simulink model "mrac_sim"  (R2023b)
settings: Solver=FixedStepDiscrete  StartTime=0.0  StopTime=6*60  FixedStep=0.1  RelTol=1e-3  EnableMultiTasking=on
undefined symbols (not defined in the file): Advantech, PCI
libraries: sldrtlib x4
settings Model: Creator=Admin  LastModifiedBy=andre
settings SolverCC: AlgebraicLoopSolver=TrustRegion
settings DataIOCC: LimitDataPoints=on  SaveFormat=Array  ReturnWorkspaceOutputs=off
settings OptimizationCC: ReuseModelBlockBuffer=off  LifeSpan=inf
settings DebuggingCC: UnconnectedInputMsg=warning  UnconnectedOutputMsg=warning  UnconnectedLineMsg=warning  SFUnexpectedBacktrackingDiag=warning  SFNoUnconditionalDefaultTransitionDiag=warning  SFExecutionAtInitializationDiag=none  ArithmeticOperatorsInVariantConditions=warning
settings HardwareCC: ProdBitPerPointer=32  ProdBitPerSizeT=32  ProdBitPerPtrDiffT=32  ProdLargestAtomicFloat=None  ProdIntDivRoundTo=Undefined  ProdEndianess=Unspecified  ProdWordSize=32  ProdHWDeviceType=32-bit Generic
settings ModelReferenceCC: PropagateSignalLabelsOutOfModel=off
settings SFSimCC: SimUseLocalCustomCode=off  CustomCodeUndefinedFunction=UseInterfaceOnly
settings RTWCC: RTWUseLocalCustomCode=off
settings CodeAppCC: StateflowObjectComments=on
settings GRTTargetCC: TargetLangStandard=C89/C90 (ANSI)
settings ConfigComp: CovMetricSettings=dw  CovSaveCumulativeToWorkspaceVar=on  CovSaveSingleToWorkspaceVar=on  CovExternalEMLEnable=off

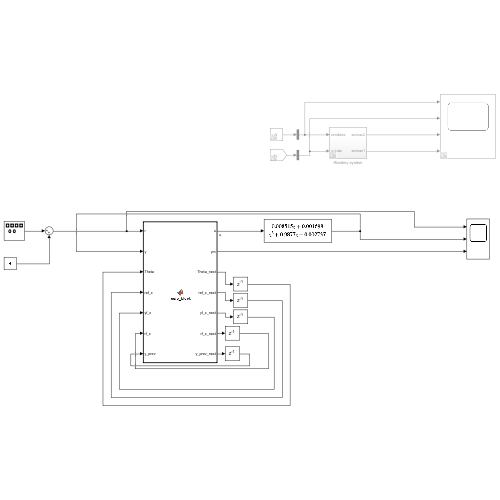
[thumbnail: Simulink's stored preview of the top-level diagram]
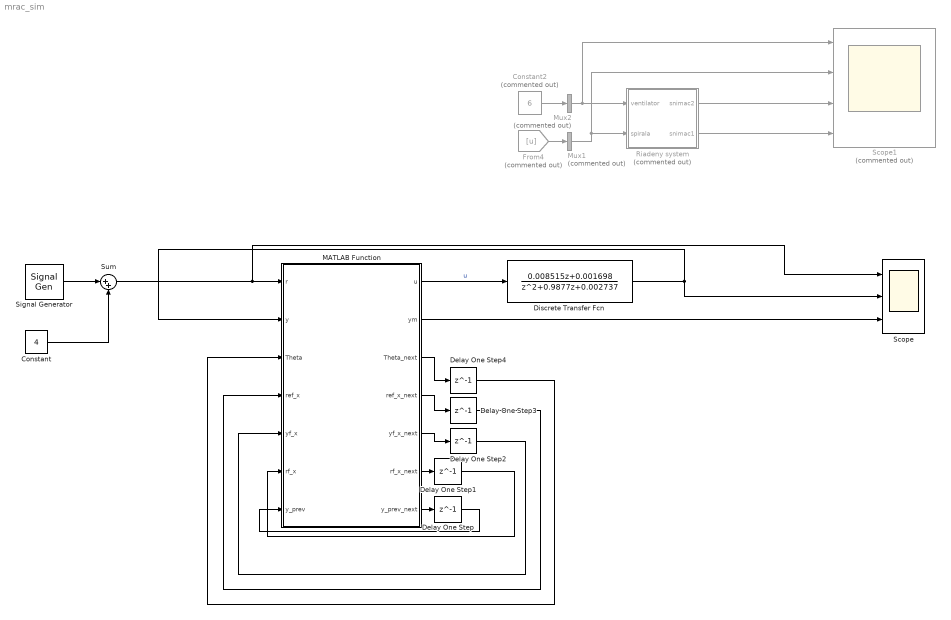
== system mrac_sim ==
  Constant : Constant  Value=4
  Constant2 : Constant  Commented=on  Value=6
  Delay One Step{,1..4} (5 alike) : Delay  DelayLength=1
  Discrete Transfer Fcn : DiscreteTransferFcn  Numerator=[0.008515 0.001698]  Denominator=[1 0.9877 0.002737]
  From4 : From  Commented=on  GotoTag=u
  MATLAB Function : MATLAB Function  TreatAsAtomicUnit=on
  Mux1 : Mux  Commented=on  Inputs=1
  Mux2 : Mux  Commented=on  Inputs=1
  Riadeny system : Subsystem  Commented=on
  Scope : Scope  NumInputPorts=3
  Scope1 : Scope  Commented=on  NumInputPorts=4
  Signal Generator : SignalGenerator  WaveForm=square  Amplitude=2  Frequency=1/50
  Sum : Sum  Inputs=|++
  wires:
  From4/1 -> Mux1/1
  Mux1/1 -> Riadeny system/2(spirala), Scope1/2
  Riadeny system/2(snimac1) -> Scope1/4
  Mux2/1 -> Riadeny system/1(ventilator), Scope1/1
  Riadeny system/1(snimac2) -> Scope1/3
  Constant2/1 -> Mux2/1
  MATLAB Function/7(y_prev_next) -> Delay One Step/1
  MATLAB Function/6(rf_x_next) -> Delay One Step1/1
  MATLAB Function/5(yf_x_next) -> Delay One Step2/1
  MATLAB Function/4(ref_x_next) -> Delay One Step3/1
  MATLAB Function/3(Theta_next) -> Delay One Step4/1
  Sum/1 -> Scope/1, MATLAB Function/1(r)
  Discrete Transfer Fcn/1 -> MATLAB Function/2(y), Scope/2
  MATLAB Function/1(u) -> Discrete Transfer Fcn/1  "u"
  Delay One Step4/1 -> MATLAB Function/3(Theta)
  Delay One Step3/1 -> MATLAB Function/4(ref_x)
  Delay One Step2/1 -> MATLAB Function/5(yf_x)
  Delay One Step1/1 -> MATLAB Function/6(rf_x)
  Delay One Step/1 -> MATLAB Function/7(y_prev)
  Signal Generator/1 -> Sum/1
  Constant/1 -> Sum/2
  MATLAB Function/2(ym) -> Scope/3

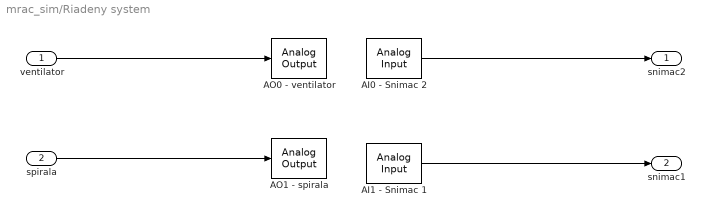
== system mrac_sim/Riadeny system ==
  ventilator : Inport
  spirala : Inport  Port=2
  AI0 - Snimac 2 : sldrtlib/Analog Input  SampleTime=0.1  MaxMissedTicks=10  ShowMissedTicks=off  YieldWhenWaiting=off  DrvName=Advantech/PCI-1711  DrvAddress=4294967295  DrvOptions=zeros(1,0)  Channels=1  RangeMode=1  VoltRange=1  DataType=1
      settings: AttributesFormatString=Advantech\nPCI-1711 [auto]
  AI1 - Snimac 1 : sldrtlib/Analog Input  SampleTime=0.1  MaxMissedTicks=10  ShowMissedTicks=off  YieldWhenWaiting=off  DrvName=Advantech/PCI-1711  DrvAddress=4294967295  DrvOptions=zeros(1,0)  Channels=2  RangeMode=1  VoltRange=1  DataType=1
      settings: AttributesFormatString=Advantech\nPCI-1711 [auto]
  AO0 - ventilator : sldrtlib/Analog Output  SampleTime=0.1  MaxMissedTicks=10  ShowMissedTicks=off  YieldWhenWaiting=off  DrvName=Advantech/PCI-1711  DrvAddress=4294967295  DrvOptions=zeros(1,0)  Channels=1  RangeMode=1  VoltRange=2  InitialValue=[]  FinalValue=[]
      settings: AttributesFormatString=Advantech\nPCI-1711 [auto]
  AO1 - spirala : sldrtlib/Analog Output  SampleTime=0.1  MaxMissedTicks=10  ShowMissedTicks=off  YieldWhenWaiting=off  DrvName=Advantech/PCI-1711  DrvAddress=4294967295  DrvOptions=zeros(1,0)  Channels=2  RangeMode=1  VoltRange=2  InitialValue=[]  FinalValue=[]
      settings: AttributesFormatString=Advantech\nPCI-1711 [auto]
  snimac2 : Outport
  snimac1 : Outport  Port=2
  wires:
  ventilator/1 -> AO0 - ventilator/1
  spirala/1 -> AO1 - spirala/1
  AI1 - Snimac 1/1 -> snimac1/1
  AI0 - Snimac 2/1 -> snimac2/1

== matlab function mrac_sim/MATLAB Function ==
  data: r input size=[1 1]; y input size=[1 1]; u output size=[1 1]; ym output size=[1 1]; Theta input size=[3 1]; ref_x input size=[2 1]; Theta_next output size=[3 1]; yf_x input size=[2 1]; rf_x input size=[2 1]; y_prev input size=[1 1]; ref_x_next output size=[2 1]; yf_x_next output size=[2 1]; rf_x_next output size=[2 1]; y_prev_next output size=[1 1]
function [u, ym, Theta_next, ref_x_next, yf_x_next, rf_x_next, y_prev_next] = mrac_block(r, y, Theta, ref_x, yf_x, rf_x, y_prev)

%constant_parameters
a0m = 1;
a1m = 5;
b0m = 1;

alpha1 = 0.6;
alpha2 = 0.001;
alpha3 = 0.005;

sign_b0 = 1;
Ts = 0.1;

A = [0,    1;
     -a0m, -a1m];

B_ref = [0;
         b0m];

B_f = [0;
       1];

%derivation

ydot = (y - y_prev)/Ts;

%outputs from current state

ym = ref_x(1);
yf = yf_x(1);
yf_s = yf_x(2);
rf = rf_x(1);

%error

e = y - ym;

%control law

omega = [y; ydot; r];
u = Theta.' * omega;

%MIT law

dTheta = -sign_b0 * e * [alpha1 * yf; alpha2 * yf_s; alpha3 * rf];
Theta_next = Theta + Ts * dTheta;

%State updates by Euler

ref_x_next = ref_x + Ts * (A * ref_x + B_ref * r);
yf_x_next = yf_x + Ts * (A * yf_x + B_f * y);
rf_x_next = rf_x + Ts * (A * rf_x + B_f * r);

%memory upfate for derivative

y_prev_next = y;

end
